simulink model "BPN_test"  (Simulink 7.4)
settings: Solver=FixedStepDiscrete  StartTime=0.0  StopTime=10.0  FixedStep=0.01  RelTol=1e-3
libraries: BPN_lib x1
settings Model: Creator=lixuying  LastModifiedBy=lixuying
settings DataIOCC: SaveFormat=StructureWithTime
settings OptimizationCC: InlineParams=on
settings DebuggingCC: SignalResolutionControl=TryResolveAll

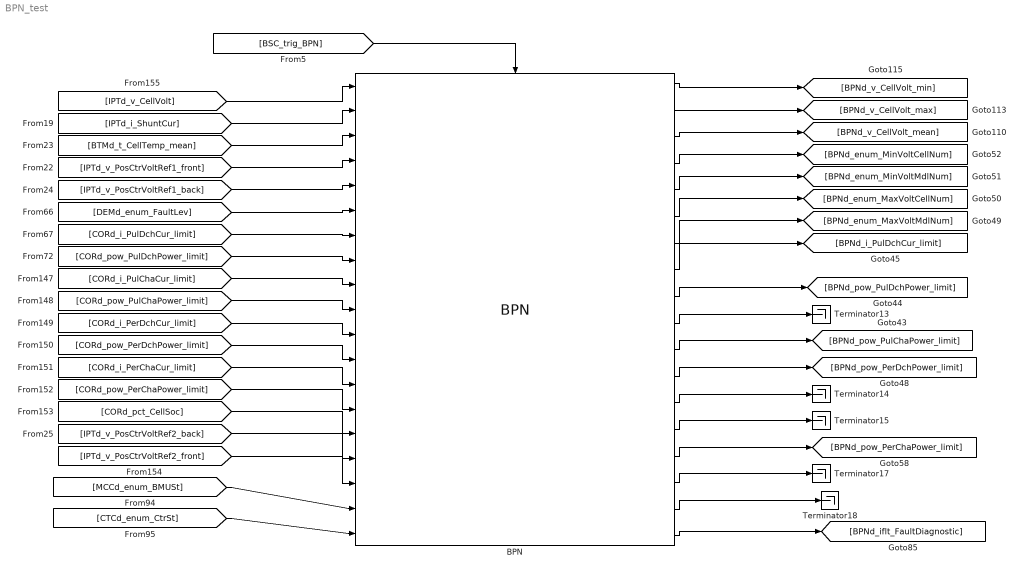
== system BPN_test ==
  BPN : BPN_lib/BPN  SystemSampleTime=-1
  Terminator{13..15,17..18} (5 alike) : Terminator
  wires:
  [BSC_trig_BPN] -> BPN/Trigger
  [IPTd_v_CellVolt] -> BPN/1
  [IPTd_i_ShuntCur] -> BPN/2
  [BTMd_t_CellTemp_mean] -> BPN/3
  [IPTd_v_PosCtrVoltRef1_front] -> BPN/4
  [IPTd_v_PosCtrVoltRef1_back] -> BPN/5
  [DEMd_enum_FaultLev] -> BPN/6
  [CORd_i_PulDchCur_limit] -> BPN/7
  [IPTd_v_PosCtrVoltRef2_back] -> BPN/16
  [CORd_pow_PulDchPower_limit] -> BPN/8
  [CORd_i_PulChaCur_limit] -> BPN/9
  [CORd_pow_PulChaPower_limit] -> BPN/10
  [CORd_i_PerDchCur_limit] -> BPN/11
  [CORd_pow_PerDchPower_limit] -> BPN/12
  [CORd_i_PerChaCur_limit] -> BPN/13
  [CORd_pow_PerChaPower_limit] -> BPN/14
  [CORd_pct_CellSoc] -> BPN/15
  [IPTd_v_PosCtrVoltRef2_front] -> BPN/17
  BPN/1 -> [BPNd_v_CellVolt_min]
  BPN/2 -> [BPNd_v_CellVolt_max]
  BPN/3 -> [BPNd_v_CellVolt_mean]
  BPN/4 -> [BPNd_enum_MinVoltCellNum]
  BPN/5 -> [BPNd_enum_MinVoltMdlNum]
  BPN/6 -> [BPNd_enum_MaxVoltCellNum]
  BPN/7 -> [BPNd_enum_MaxVoltMdlNum]
  BPN/8 -> [BPNd_i_PulDchCur_limit]
  BPN/9 -> [BPNd_pow_PulDchPower_limit]
  BPN/10 -> Terminator13/1
  BPN/11 -> [BPNd_pow_PulChaPower_limit]
  BPN/12 -> [BPNd_pow_PerDchPower_limit]
  BPN/13 -> Terminator14/1
  BPN/14 -> Terminator15/1
  BPN/15 -> [BPNd_pow_PerChaPower_limit]
  BPN/16 -> Terminator17/1
  BPN/17 -> Terminator18/1
  BPN/18 -> [BPNd_iflt_FaultDiagnostic]
  [MCCd_enum_BMUSt] -> BPN/18
  [CTCd_enum_CtrSt] -> BPN/19
